simulink model "template_hardware_digital_sim"  (R2021b)
settings: Solver=FixedStepAuto  StartTime=0.0  StopTime=60  FixedStep=1e-3  RelTol=1e-3  EnableMultiTasking=on
undefined symbols (not defined in the file or in its folder): K_d, K_d_new
libraries: cstblocks x3, qube2servo x3
settings Model: SimulationMode=external  ExtModeTrigDuration=5000  Creator=MLevis  LastModifiedBy=12288
settings SolverCC: AlgebraicLoopSolver=TrustRegion  PositivePriorityOrder=on
settings DataIOCC: LimitDataPoints=on  SaveFormat=Array  SignalLoggingSaveFormat=ModelDataLogs  ReturnWorkspaceOutputs=off
settings OptimizationCC: BooleanDataType=off  OptimizeBlockIOStorage=off  BufferReuse=off  GlobalBufferReuse=off  ExpressionFolding=off  ExpressionDepthLimit=2147483647  LocalBlockOutputs=off  InitFltsAndDblsToZero=on  LifeSpan=inf  OptimizeDataStoreBuffers=off  BusAssignmentInplaceUpdate=off
settings DebuggingCC: SaveWithParameterizedLinksMsg=none  UnderspecifiedInitializationDetection=Classic  MergeDetectMultiDrivingBlocksExec=none  SignalResolutionControl=TryResolveAllWithWarning  MultiTaskDSMMsg=warning  MultiTaskCondExecSysMsg=none  FcnCallInpInsideContextMsg=warning  StateNameClashWarn=warning  SFUnexpectedBacktrackingDiag=warning  SFNoUnconditionalDefaultTransitionDiag=warning  SFExecutionAtInitializationDiag=none  SFMachineParentedDataDiag=warning  ArithmeticOperatorsInVariantConditions=warning
settings HardwareCC: ProdBitPerPointer=32  ProdBitPerSizeT=32  ProdBitPerPtrDiffT=32  ProdLargestAtomicFloat=None  ProdIntDivRoundTo=Undefined  ProdEndianess=Unspecified  ProdWordSize=32  ProdHWDeviceType=32-bit Generic  TargetHWDeviceType=32-bit Generic
settings ModelReferenceCC: PropagateSignalLabelsOutOfModel=off
settings SFSimCC: SimUseLocalCustomCode=off  SimParseCustomCode=off  CustomCodeUndefinedFunction=UseInterfaceOnly
settings RTWCC: Description=QUARC Win64 Target  SystemTargetFile=quarc_win64.tlc  TemplateMakefile=quarc_default_tmf  RTWUseLocalCustomCode=off
settings CodeAppCC: StateflowObjectComments=on
settings STFCustomTargetCC: TargetPreCompLibLocation=C:\PROGRA~3\QUARC\lib\2017a\win64\release  ConcurrentExecutionCompliant=on  SystemTargetFile=quarc_win64.tlc
settings GRTTargetCC: TargetPreCompLibLocation=C:\PROGRA~3\QUARC\lib\2017a\win64\release  TargetLangStandard=C89/C90 (ANSI)  ParMdlRefBuildCompliant=off  CompOptLevelCompliant=off  CombineOutputUpdateFcns=off  MatFileLogging=off  CPPClassGenCompliant=off  GRTInterface=on  UseToolchainInfoCompliant=off  ExtMode=on  ExtModeMexFile=quarc_comm
settings ConfigComp: CovMetricSettings=dw  CovSaveCumulativeToWorkspaceVar=on  CovSaveSingleToWorkspaceVar=on  CovExternalEMLEnable=off  CovSFcnEnable=off

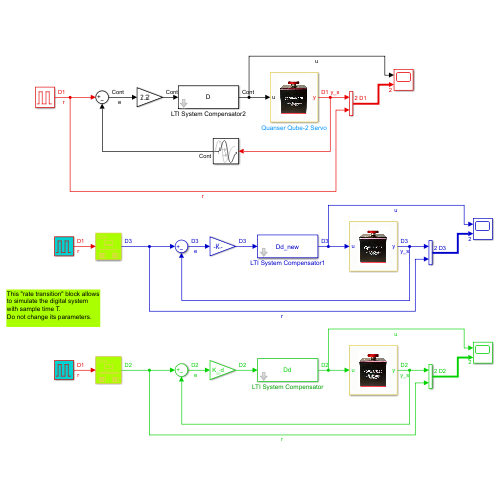
[thumbnail: Simulink's stored preview of the top-level diagram]
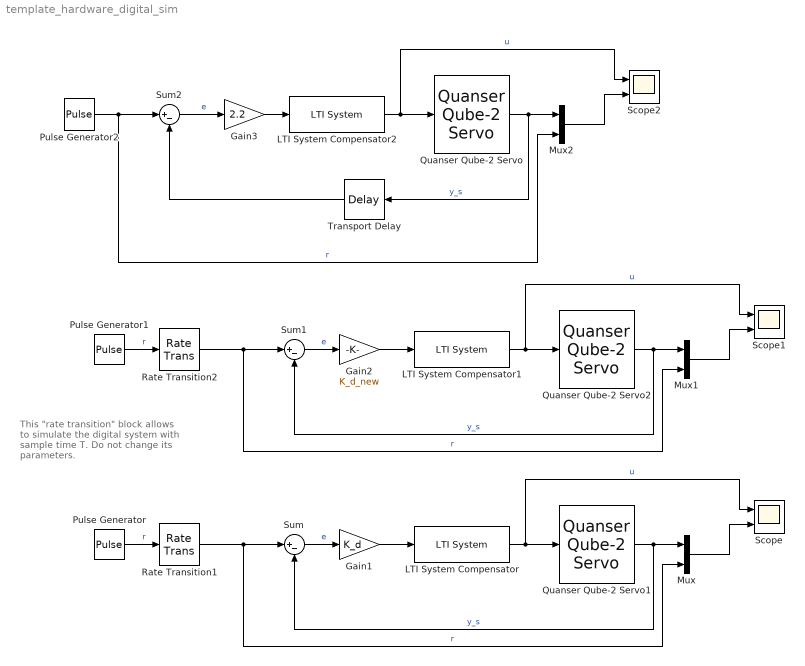
== system template_hardware_digital_sim ==
  note: This "rate transition" block allows to simulate the digital system with sample time T.
      | Do not change its parameters.
  Gain1 : Gain  Gain=K_d
  Gain2 : Gain  Gain=K_d_new
  Gain3 : Gain  Gain=2.2
  LTI System Compensator : cstblocks/LTI System  sys=Dd  IC=[]
  LTI System Compensator1 : cstblocks/LTI System  sys=Dd_new  IC=[]
  LTI System Compensator2 : cstblocks/LTI System  sys=D  IC=[]
  Mux : Mux  Inputs=2
  Mux1 : Mux  Inputs=2
  Mux2 : Mux  Inputs=2
  Pulse Generator : DiscretePulseGenerator  PulseType=Time based  Period=8  PulseWidth=50
  Pulse Generator1 : DiscretePulseGenerator  PulseType=Time based  Period=8  PulseWidth=50
  Pulse Generator2 : DiscretePulseGenerator  PulseType=Time based  Period=10  PulseWidth=50
  Quanser Qube-2 Servo : qube2servo/Quanser Qube-2 Servo  SystemSampleTime=-1  VariantActivationTime=update diagram  Latency=0  AutoFrameSizeCalculation=off
  Quanser Qube-2 Servo1 : qube2servo/Quanser Qube-2 Servo  SystemSampleTime=-1  VariantActivationTime=update diagram  Latency=0  AutoFrameSizeCalculation=off
  Quanser Qube-2 Servo2 : qube2servo/Quanser Qube-2 Servo  SystemSampleTime=-1  VariantActivationTime=update diagram  Latency=0  AutoFrameSizeCalculation=off
  Rate Transition1 : RateTransition
  Rate Transition2 : RateTransition
  Scope : Scope  NumInputPorts=2
  Scope1 : Scope  NumInputPorts=2
  Scope2 : Scope  NumInputPorts=2
  Sum : Sum  Inputs=|+-
  Sum1 : Sum  Inputs=|+-
  Sum2 : Sum  Inputs=|+-
  Transport Delay : TransportDelay  DelayTime=0
  wires:
  Pulse Generator/1 -> Rate Transition1/1  "r"
  Rate Transition1/1 -> Mux/2, Sum/1  "r"
  Sum/1 -> Gain1/1  "e"
  Mux/1 -> Scope/2
  Quanser Qube-2 Servo1/1 -> Sum/2, Mux/1  "y_s"
  Gain1/1 -> LTI System Compensator/1
  LTI System Compensator/1 -> Quanser Qube-2 Servo1/1, Scope/1  "u"
  Rate Transition2/1 -> Mux1/2, Sum1/1  "r"
  Pulse Generator1/1 -> Rate Transition2/1  "r"
  LTI System Compensator1/1 -> Quanser Qube-2 Servo2/1, Scope1/1  "u"
  Gain2/1 -> LTI System Compensator1/1
  Mux1/1 -> Scope1/2
  Sum1/1 -> Gain2/1  "e"
  Quanser Qube-2 Servo2/1 -> Sum1/2, Mux1/1  "y_s"
  Gain3/1 -> LTI System Compensator2/1
  Mux2/1 -> Scope2/2
  Pulse Generator2/1 -> Mux2/2, Sum2/1  "r"
  LTI System Compensator2/1 -> Quanser Qube-2 Servo/1, Scope2/1  "u"
  Quanser Qube-2 Servo/1 -> Mux2/1, Transport Delay/1  "y_s"
  Transport Delay/1 -> Sum2/2
  Sum2/1 -> Gain3/1  "e"
